simulink model "SB12_reuse_done"  (R2024b)
settings: Solver=ode45  StartTime=0.0  StopTime=6  MaxStep=0.01  RelTol=1e-3
settings Model: Creator=admin  LastModifiedBy=admin

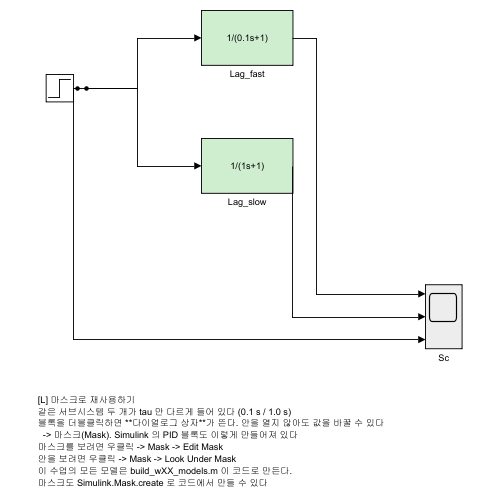
[thumbnail: Simulink's stored preview of the top-level diagram]
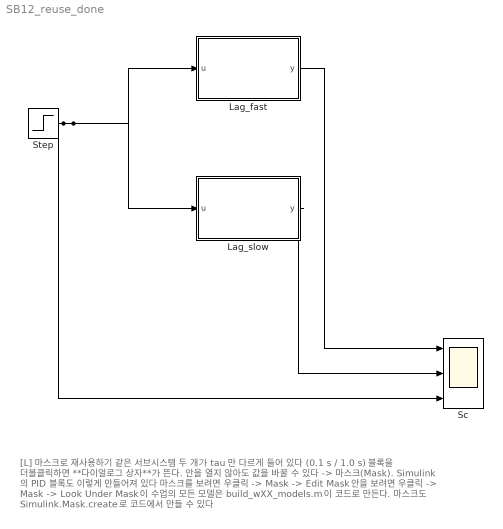
== system SB12_reuse_done ==
  note: [L] 마스크로 재사용하기
      | 같은 서브시스템 두 개가 tau 만 다르게 들어 있다 (0.1 s / 1.0 s)
      | 블록을 더블클릭하면 **다이얼로그 상자**가 뜬다. 안을 열지 않아도 값을 바꿀 수 있다
      |   -> 마스크(Mask). Simulink 의 PID 블록도 이렇게 만들어져 있다
      | 마스크를 보려면 우클릭 -> Mask -> Edit Mask
      | 안을 보려면 우클릭 -> Mask -> Look Under Mask
      | 이 수업의 모든 모델은 build_wXX_models.m 이 코드로 만든다.
      | 마스크도 Simulink.Mask.create 로 코드에서 만들 수 있다
  Lag_fast : Subsystem  mask{tau=0.1}
      mask prompts: tau "시상수 tau [s]"
      mask help:
      | 1차 지연.  dy/dt = (u - y)/tau
      | 5주차 모터 응답 모델과 같은 식이다.
      mask Display: disp(sprintf('1/(%gs+1)', tau))
  Lag_slow : Subsystem  mask{tau=1.0}
      mask prompts: tau "시상수 tau [s]"
      mask help:
      | 1차 지연.  dy/dt = (u - y)/tau
      | 5주차 모터 응답 모델과 같은 식이다.
      mask Display: disp(sprintf('1/(%gs+1)', tau))
  Sc : Scope  NumInputPorts=3
  Step : Step  SampleTime=0
  wires:
  Step/1 -> Lag_fast/1(u), Lag_slow/1(u), Sc/3
  Lag_slow/1(y) -> Sc/2
  Lag_fast/1(y) -> Sc/1

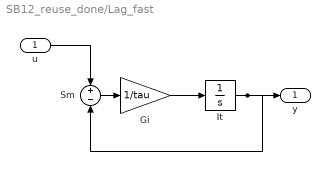
== system SB12_reuse_done/Lag_fast ==
  u : Inport
  Gi : Gain  Gain=1/tau
  It : Integrator
  Sm : Sum  Inputs=+-
  y : Outport
  wires:
  u/1 -> Sm/1
  Sm/1 -> Gi/1
  It/1 -> Sm/2, y/1
  Gi/1 -> It/1

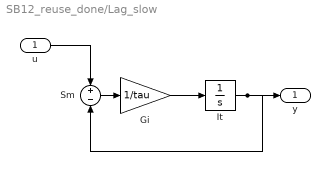
== system SB12_reuse_done/Lag_slow ==
  u : Inport
  Gi : Gain  Gain=1/tau
  It : Integrator
  Sm : Sum  Inputs=+-
  y : Outport
  wires:
  It/1 -> Sm/2, y/1
  u/1 -> Sm/1
  Sm/1 -> Gi/1
  Gi/1 -> It/1
